simulink model "test_loopback_buf"  (Simulink 6.2)
settings: Solver=ode45  StartTime=0.0  StopTime=4000  RelTol=1e-3
undefined symbols (not defined in the file): Down, Up
libraries: xbsIndex_r3 x1383, xps_library x52, casper_library x37
(part 5 of 8)

== system test_loopback_buf/xaui_buffer_old1 ==
  note: MUX TWO PACKET STREAMS
      | Incomming data is buffered and only stored if it is commited (valid EOF).
      | If a discard command is received, the data is flushed.
  note: THE ACK LINE MUST REMAIN HIGH EVEN WHEN VALID GOES LOW FOR FULL-SPEED READOUT.
      |
      | This is fine for the intended purpose:
      | We read out a full packet at a time, ensuring that ack stays high until EOF is received.
      |
      | this is also important to ensure that the wrong IP address is not used
      | (there is a one-clock delay to fetch the next IP)
  note: PACKET LENGTH SHOULD NOT BE LESS THAN 3 WORDS
  d_in : Inport  Port=1  LatchInput=off
  valid_in : Inport  Port=2  LatchInput=off
  dest_ip_0 : Inport  Port=3  LatchInput=off
  eof_in : Inport  Port=4  LatchInput=off
  discard_in : Inport  Port=5  LatchInput=off
  ack_out : Inport  Port=6  LatchInput=off
  Concat : xbsIndex_r3/Concat  num_inputs=2  explicit_period=off  period=1  dbl_ovrd=off
  Concat3 : xbsIndex_r3/Concat  num_inputs=2  explicit_period=off  period=1  dbl_ovrd=off
  Concat_status : xbsIndex_r3/Concat  num_inputs=4  explicit_period=on  period=1  dbl_ovrd=off
  Constant13 : xbsIndex_r3/Constant  const=0  equ=P=C  arith_type=Boolean  n_bits=1  bin_pt=0  opselect=C  inp2=PCIN>>17  opr=+  inp1=P  carry=CIN  iostate=0  explicit_period=on  period=1  dbl_ovrd=off
  Constant7 : xbsIndex_r3/Constant  const=0  equ=P=C  arith_type=Unsigned  n_bits=32-9  bin_pt=0  opselect=C  inp2=PCIN>>17  opr=+  inp1=P  carry=CIN  iostate=0  explicit_period=on  period=1  dbl_ovrd=off
  Constant9 : xbsIndex_r3/Constant  const=0  equ=P=C  arith_type=Boolean  n_bits=1  bin_pt=0  opselect=C  inp2=PCIN>>17  opr=+  inp1=P  carry=CIN  iostate=0  explicit_period=on  period=1  dbl_ovrd=off
  Convert{,2..4} (4 alike) : xbsIndex_r3/Convert  arith_type=Boolean  n_bits=8  bin_pt=6  quantization=Truncate  overflow=Wrap  latency=0  explicit_period=on  period=1  dbl_ovrd=off  show_param=off  inserted_by_tool=off  pipeline=off
      settings: xl_area=[0, 0, 0, 0, 0, 0, 0]
  Convert{1,5,8..9} (4 alike) : xbsIndex_r3/Convert  arith_type=Unsigned  n_bits=1  bin_pt=0  quantization=Truncate  overflow=Wrap  latency=0  explicit_period=off  period=1  dbl_ovrd=off  show_param=off  inserted_by_tool=off  pipeline=off
      settings: xl_area=[0, 0, 0, 0, 0, 0, 0]
  Gateway Out{1..3,6..8,14,22..25,27..31,39..42} (20 alike) : xbsIndex_r3/Gateway Out  output_type=Double  nbits=8  bin_pt=6  arith_type=Boolean  quantization=Truncate  overflow=Wrap  hdl_port=on  timing_constraint=None  locs_specified=off  LOCs={}  needs_fixed_name=off  show_param=off
      settings: xl_area=[0, 0, 0, 0, 0, 0, 0]
  Inverter4 : xbsIndex_r3/Inverter  latency=0  explicit_period=off  period=1  en=off  dbl_ovrd=off  show_param=off
      settings: xl_area=[0, 0, 0, 0, 0, 0, 0]
  Reinterpret : xbsIndex_r3/Reinterpret  force_arith_type=on  arith_type=Unsigned  force_bin_pt=on  bin_pt=0  force_valid=on
  buf_data3 : xbsIndex_r3/Slice  mode=Lower Bit Location + Width  nbits=64  bit1=33  base1=LSB of Input  bit0=0  base0=LSB of Input  boolean_output=off  explicit_period=off  period=1  dbl_ovrd=off
  buf_eof1 : xbsIndex_r3/Slice  mode=Upper Bit Location + Width  nbits=1  bit1=64  base1=LSB of Input  bit0=0  base0=LSB of Input  boolean_output=on  explicit_period=off  period=1  dbl_ovrd=off
  buf_eof3 : xbsIndex_r3/Slice  mode=Upper Bit Location + Width  nbits=1  bit1=64  base1=LSB of Input  bit0=0  base0=LSB of Input  boolean_output=on  explicit_period=off  period=1  dbl_ovrd=off
  commit : xbsIndex_r3/Logical  logical_function=AND  inputs=2  precision=Full  arith_type=Unsigned  n_bits=8  bin_pt=2  align_bp=on  latency=0  explicit_period=off  period=1  en=off  dbl_ovrd=off  show_param=off
      settings: xl_area=[0, 0, 0, 0, 0, 0, 0]
  data_FWFT : Subsystem  mask{depth_bits=depth_data_bits}
      mask prompts: depth_bits "Fifo Depth (2^?):"
      mask help: A rollback fifo behaves as a normal fifo, except that data which are written in have to be "committed" before they become available for readout. Moreover, any data which are written in and have not been committed can be "discarded", and will never be made available for readout.
      mask init:
      | fmtstr = sprintf('Depth: %d', 2^depth_bits);
      | set_param(gcb, 'AttributesFormatString', fmtstr);
      settings: AttributesFormatString=Depth: 1024
  data_debug : Scope  NumInputPorts=10
      settings: YMin=12000~0~9500~0~15500~0~0~-5~-5~-5  YMax=13300~1~10500~1~17250~1~1~5~5~5  SaveName=ScopeData8
  fifo_empty : xbsIndex_r3/Logical  logical_function=AND  inputs=2  precision=Full  arith_type=Unsigned  n_bits=8  bin_pt=2  align_bp=on  latency=0  explicit_period=off  period=1  en=off  dbl_ovrd=off  show_param=off
      settings: xl_area=[0, 0, 0, 0, 0, 0, 0]
  fifo_full : xbsIndex_r3/Logical  logical_function=OR  inputs=2  precision=Full  arith_type=Unsigned  n_bits=8  bin_pt=2  align_bp=on  latency=0  explicit_period=off  period=1  en=off  dbl_ovrd=off  show_param=off
      settings: xl_area=[0, 0, 0, 0, 0, 0, 0]
  ip_debug : Scope  NumInputPorts=6
      settings: YMin=100~0~0~100~0~-5  YMax=103~1~1~103~1~5  SaveName=ScopeData9
  ip_fifo : Subsystem  mask{depth_bits=depth_hdr_bits}
      mask prompts: depth_bits "Fifo Depth (2^?):"
      mask help: A rollback fifo behaves as a normal fifo, except that data which are written in have to be "committed" before they become available for readout. Moreover, any data which are written in and have not been committed can be "discarded", and will never be made available for readout.
      mask init:
      | fmtstr = sprintf('Depth: %d', 2^depth_bits);
      | set_param(gcb, 'AttributesFormatString', fmtstr);
      settings: AttributesFormatString=Depth: 256
  overflow_cnt : xps_library/software register  Tag=xps:sw_reg  io_dir=To Processor  arith_type=Unsigned  bitwidth=32  bin_pt=0  sample_period=1  gw_name=test_loopback_buf_xaui_buffer_old1_overflow_cnt_user_data_in
  overflows : xbsIndex_r3/Counter  cnt_type=Free Running  n_bits=32  bin_pt=0  arith_type=Unsigned  start_count=0  cnt_to=Inf  cnt_by_val=1  operation=Up  explicit_period=off  period=1  load_pin=off  rst=off  en=on  dbl_ovrd=off  show_param=off  use_rpm=on  gen_core=off
      settings: xl_area=[0, 0, 0, 0, 0, 0, 0]
  status : xps_library/software register  Tag=xps:sw_reg  io_dir=To Processor  arith_type=Unsigned  bitwidth=32  bin_pt=0  sample_period=1  gw_name=test_loopback_buf_xaui_buffer_old1_status_user_data_in
  status1 : Scope  NumInputPorts=4
      settings: YMin=-1~-1~-1~-1  YMax=1~1~1~1  SaveName=ScopeData6
  valid_eof_0 : xbsIndex_r3/Logical  logical_function=AND  inputs=2  precision=Full  arith_type=Unsigned  n_bits=8  bin_pt=2  align_bp=on  latency=0  explicit_period=on  period=1  en=off  dbl_ovrd=off  show_param=off
      settings: xl_area=[0, 0, 0, 0, 0, 0, 0]
  data : Outport
  valid : Outport  Port=2
  ip_addr : Outport  Port=3
  eof : Outport  Port=4
  discard : Outport  Port=5
  buffer_overflow : Outport  Port=6
  buffer_empty : Outport  Port=7
  ack_in : Outport  Port=8
  status_out : Outport  Port=9
  wires:
  Constant13/1 -> discard/1
  fifo_full/1 -> buffer_overflow/1, overflows/1
  fifo_empty/1 -> buffer_empty/1
  [ip_empty] -> fifo_empty/1
  [data_empty] -> fifo_empty/2
  [ip_full] -> fifo_full/1
  [data_full] -> fifo_full/2
  [ip_full] -> Convert1/1, Gateway Out7/1
  [data_full] -> Gateway Out8/1, Convert5/1
  [ip_empty] -> Convert8/1, Gateway Out6/1
  [data_empty] -> Convert9/1, Gateway Out14/1
  Concat_status/1 -> Concat3/2, status_out/1
  Concat3/1 -> status/1
  Constant7/1 -> Concat3/1
  discard_in/1 -> Convert3/1
  Concat/1 -> data_FWFT/1(din)
  data_FWFT/4(full) -> [data_full]
  ip_fifo/3(full) -> [ip_full]
  commit/1 -> ip_fifo/3(commit), ip_fifo/2(we), [ip_commit]
  d_in/1 -> Reinterpret/1
  valid_in/1 -> Convert/1
  dest_ip_0/1 -> ip_fifo/1(din), [ip_in]
  eof_in/1 -> Convert2/1
  data_FWFT/3(wr_ack) -> ack_in/1
  ip_fifo/4(empty) -> [ip_empty]
  Inverter4/1 -> commit/2
  valid_eof_0/1 -> Concat/1, [in_valid_eof], data_FWFT/3(commit)
  data_FWFT/1(dout) -> buf_eof1/1, buf_eof3/1, buf_data3/1
  data_FWFT/2(valid) -> valid/1, [v_out]
  ip_fifo/1(dout) -> ip_addr/1, [ip_out]
  Constant9/1 -> ip_fifo/4(discard)
  overflows/1 -> overflow_cnt/1
  Gateway Out24/1 -> data_debug/1
  Gateway Out22/1 -> data_debug/2
  Gateway Out23/1 -> data_debug/3
  Gateway Out25/1 -> data_debug/4
  Gateway Out29/1 -> ip_debug/1
  Gateway Out27/1 -> ip_debug/2
  Gateway Out28/1 -> ip_debug/3
  Gateway Out30/1 -> ip_debug/4
  Gateway Out31/1 -> ip_debug/5
  Gateway Out39/1 -> data_debug/5
  Gateway Out41/1 -> data_debug/6
  Gateway Out40/1 -> data_debug/7
  Gateway Out42/1 -> ip_debug/6
  data_FWFT/5(empty) -> [data_empty]
  buf_data3/1 -> data/1, [d_out]
  buf_eof3/1 -> eof/1, [eof_out]
  [in_valid_eof] -> commit/1
  Gateway Out7/1 -> status1/1
  Gateway Out8/1 -> status1/2
  Gateway Out6/1 -> status1/3
  Gateway Out14/1 -> status1/4
  Convert1/1 -> Concat_status/1
  Convert5/1 -> Concat_status/2
  Convert8/1 -> Concat_status/3
  Convert9/1 -> Concat_status/4
  Gateway Out1/1 -> data_debug/8
  [ip_out] -> Gateway Out1/1
  [eof_out] -> Gateway Out40/1
  [v_out] -> Gateway Out41/1
  [d_out] -> Gateway Out39/1
  [ip_in] -> Gateway Out25/1
  [d_in] -> Gateway Out24/1
  [v_in] -> Gateway Out22/1
  [in_valid_eof] -> Gateway Out23/1
  [ip_in] -> Gateway Out29/1
  [ip_out] -> Gateway Out30/1
  [eof_out] -> Gateway Out31/1
  ack_out/1 -> Convert4/1
  [data_ack] -> Gateway Out42/1
  [ip_commit] -> Gateway Out27/1
  [data_full] -> Inverter4/1
  [ip_fetch] -> Gateway Out28/1
  [data_ack] -> data_FWFT/5(ack)
  Gateway Out2/1 -> data_debug/9
  [data_ack] -> Gateway Out2/1
  buf_eof1/1 -> [ip_fetch]
  [ip_fetch] -> ip_fifo/5(fetch)
  Reinterpret/1 -> Concat/2, [d_in]
  Convert/1 -> valid_eof_0/1, data_FWFT/2(we), [v_in]
  Convert2/1 -> valid_eof_0/2
  Convert3/1 -> data_FWFT/4(discard)
  Convert4/1 -> [data_ack]
  Gateway Out3/1 -> data_debug/10
  [data_full] -> Gateway Out3/1

== system test_loopback_buf/loopback/fwft_fifo ==
  din : Inport  Port=1  LatchInput=off
  we : Inport  Port=2  LatchInput=off
  ack : Inport  Port=3  LatchInput=off
  Convert : xbsIndex_r3/Convert  Orientation=left  arith_type=Boolean  n_bits=1  bin_pt=0  quantization=Truncate  overflow=Wrap  latency=0  explicit_period=off  period=1  dbl_ovrd=off  show_param=off  inserted_by_tool=off  pipeline=off
      settings: xl_area=[0, 0, 0, 0, 0, 0, 0]
  FIFO : xbsIndex_r3/FIFO  depth=256  percent_nbits=1  store_only_valid=on  init_zero=on  explicit_period=off  period=1  rst=off  en=off  use_almost_empty=off  almost_empty_offset=6  use_almost_full=off  almost_full_offset=6  dbl_ovrd=off  show_param=off  mem_type=Block RAM  gen_core=off
      settings: xl_area=[0, 0, 0, 0, 0, 0, 0]
  Inverter1 : xbsIndex_r3/Inverter  latency=0  explicit_period=off  period=1  en=off  dbl_ovrd=off  show_param=off
      settings: xl_area=[0, 0, 0, 0, 0, 0, 0]
  Logical1 : xbsIndex_r3/Logical  logical_function=OR  inputs=2  precision=Full  arith_type=Unsigned  n_bits=8  bin_pt=2  align_bp=on  latency=0  explicit_period=off  period=1  en=off  dbl_ovrd=off  show_param=off
      settings: xl_area=[0, 0, 0, 0, 0, 0, 0]
  Register2 : xbsIndex_r3/Register  init=0  reg_only_valid=off  explicit_period=on  period=1  rst=off  en=on  out_en=off  dbl_ovrd=off  show_param=off
      settings: xl_area=[0, 0, 0, 0, 0, 0, 0]
  dout : Outport
  valid : Outport  Port=2
  wires:
  din/1 -> FIFO/1
  we/1 -> FIFO/2
  FIFO/1 -> dout/1
  FIFO/2 -> Register2/1
  Logical1/1 -> FIFO/3, Register2/2
  ack/1 -> Logical1/1
  Register2/1 -> Convert/1, Inverter1/1
  Convert/1 -> Logical1/2
  Inverter1/1 -> valid/1

== system test_loopback_buf/loopback/rollback_fifo ==
  din : Inport  Port=1  LatchInput=off
  we : Inport  Orientation=left  Port=2  LatchInput=off
  commit : Inport  Port=3  LatchInput=off
  discard : Inport  Port=4  LatchInput=off
  re : Inport  Port=5  LatchInput=off
  Constant5 : xbsIndex_r3/Constant  const=0  equ=P=C  arith_type=Boolean  n_bits=1  bin_pt=0  opselect=C  inp2=PCIN>>17  opr=+  inp1=P  carry=CIN  iostate=0  explicit_period=on  period=1  dbl_ovrd=off
  Delay1 : xbsIndex_r3/Delay  latency=1  reg_retiming=off  explicit_period=off  period=1  en=off  accept_only_valid=off  init_zero=on  dbl_ovrd=off  show_param=off
      settings: xl_area=[0, 0, 0, 0, 0, 0, 0]
  Dual Port RAM : xbsIndex_r3/Dual Port RAM  depth=2^depth_bits  initVector=0  write_mode_A=Read Before Write  write_mode_B=Read Before Write  latency=1  mem_collision=off  init_zero=on  explicit_period=off  period=1  dbl_ovrd=off  rst_a=off  init_a=0  rst_b=off  init_b=0  show_param=off  distributed_mem=off  use_rpm=off  gen_core=off
      settings: xl_area=[0, 0, 0, 0, 0, 0, 0]
  Inverter1 : xbsIndex_r3/Inverter  latency=0  explicit_period=off  period=1  en=off  dbl_ovrd=off  show_param=off
      settings: xl_area=[0, 0, 0, 0, 0, 0, 0]
  Inverter2 : xbsIndex_r3/Inverter  Orientation=up  latency=0  explicit_period=off  period=1  en=off  dbl_ovrd=off  show_param=off
      settings: xl_area=[0, 0, 0, 0, 0, 0, 0]
  Logical1 : xbsIndex_r3/Logical  logical_function=AND  inputs=2  precision=Full  arith_type=Unsigned  n_bits=8  bin_pt=2  align_bp=on  latency=0  explicit_period=off  period=1  en=off  dbl_ovrd=off  show_param=off
      settings: xl_area=[0, 0, 0, 0, 0, 0, 0]
  Logical3 : xbsIndex_r3/Logical  Orientation=left  logical_function=AND  inputs=2  precision=Full  arith_type=Unsigned  n_bits=8  bin_pt=2  align_bp=on  latency=0  explicit_period=off  period=1  en=off  dbl_ovrd=off  show_param=off
      settings: xl_area=[0, 0, 0, 0, 0, 0, 0]
  Logical4 : xbsIndex_r3/Logical  logical_function=AND  inputs=2  precision=Full  arith_type=Unsigned  n_bits=8  bin_pt=2  align_bp=on  latency=0  explicit_period=off  period=1  en=off  dbl_ovrd=off  show_param=off
      settings: xl_area=[0, 0, 0, 0, 0, 0, 0]
  Logical5 : xbsIndex_r3/Logical  logical_function=XOR  inputs=2  precision=Full  arith_type=Unsigned  n_bits=8  bin_pt=2  align_bp=on  latency=0  explicit_period=off  period=1  en=off  dbl_ovrd=off  show_param=off
      settings: xl_area=[0, 0, 0, 0, 0, 0, 0]
  Logical6 : xbsIndex_r3/Logical  logical_function=AND  inputs=2  precision=Full  arith_type=Unsigned  n_bits=8  bin_pt=2  align_bp=on  latency=0  explicit_period=off  period=1  en=off  dbl_ovrd=off  show_param=off
      settings: xl_area=[0, 0, 0, 0, 0, 0, 0]
  Relational1 : xbsIndex_r3/Relational  mode=a=b  latency=0  explicit_period=on  period=1  en=off  dbl_ovrd=off  show_param=off
      settings: xl_area=[0, 0, 0, 0, 0, 0, 0]
  Relational2 : xbsIndex_r3/Relational  mode=a=b  latency=0  explicit_period=on  period=1  en=off  dbl_ovrd=off  show_param=off
      settings: xl_area=[0, 0, 0, 0, 0, 0, 0]
  Slice : xbsIndex_r3/Slice  mode=Two Bit Locations  nbits=1  bit1=-1  base1=MSB of Input  bit0=0  base0=LSB of Input  boolean_output=off  explicit_period=off  period=1  dbl_ovrd=off
  Slice1 : xbsIndex_r3/Slice  mode=Upper Bit Location + Width  nbits=1  bit1=0  base1=MSB of Input  bit0=0  base0=LSB of Input  boolean_output=on  explicit_period=off  period=1  dbl_ovrd=off
  Slice2 : xbsIndex_r3/Slice  mode=Two Bit Locations  nbits=1  bit1=-1  base1=MSB of Input  bit0=0  base0=LSB of Input  boolean_output=off  explicit_period=off  period=1  dbl_ovrd=off
  Slice3 : xbsIndex_r3/Slice  mode=Upper Bit Location + Width  nbits=1  bit1=0  base1=MSB of Input  bit0=0  base0=LSB of Input  boolean_output=on  explicit_period=off  period=1  dbl_ovrd=off
  rd_cnt : xbsIndex_r3/Counter  cnt_type=Free Running  n_bits=depth_bits + 1  bin_pt=0  arith_type=Unsigned  start_count=0  cnt_to=Inf  cnt_by_val=1  operation=Up  explicit_period=on  period=1  load_pin=off  rst=off  en=on  dbl_ovrd=off  show_param=off  use_rpm=on  gen_core=off
      settings: xl_area=[0, 0, 0, 0, 0, 0, 0]
  set_cnt : Subsystem
  dout : Outport
  valid : Outport  Port=2
  wr_ack : Outport  Orientation=left  Port=3
  full : Outport  Port=4
  empty : Outport  Port=5
  wires:
  Relational2/1 -> Logical1/1
  Logical6/1 -> Inverter2/1, full/1
  Logical5/1 -> Logical6/1
  Relational1/1 -> Logical6/2
  Slice1/1 -> Logical5/2
  Slice3/1 -> Logical5/1
  Slice2/1 -> Relational1/1, Dual Port RAM/1
  din/1 -> Dual Port RAM/2, Dual Port RAM/5
  Slice/1 -> Relational1/2, Dual Port RAM/4
  set_cnt/2(cnt) -> Slice2/1, Slice3/1
  set_cnt/1(set_cnt) -> Relational2/1
  rd_cnt/1 -> Relational2/2, Slice1/1, Slice/1
  commit/1 -> set_cnt/1(set)
  Inverter2/1 -> Logical1/2, Logical3/1
  we/1 -> Logical3/2
  Logical3/1 -> wr_ack/1, Dual Port RAM/3, set_cnt/3(en)
  discard/1 -> set_cnt/2(undo)
  Constant5/1 -> Dual Port RAM/6
  Dual Port RAM/2 -> dout/1
  Logical1/1 -> Inverter1/1, empty/1
  Inverter1/1 -> Logical4/2
  re/1 -> Logical4/1
  Logical4/1 -> rd_cnt/1, Delay1/1
  Delay1/1 -> valid/1

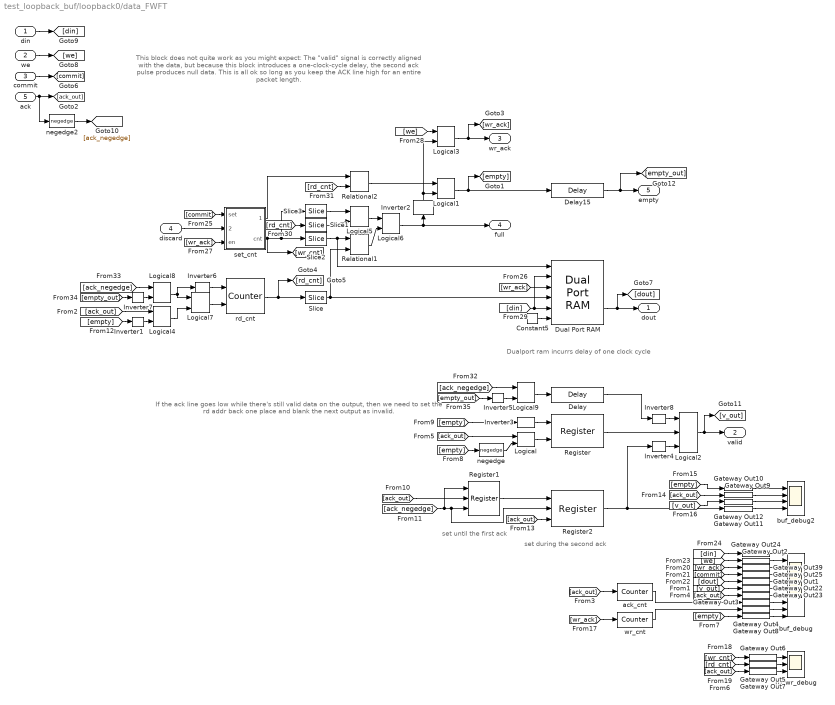
== system test_loopback_buf/loopback0/data_FWFT ==
  note: This block does not quite work as you might expect:
      | The "valid" signal is correctly aligned with the data,
      | but because this block introduces a one-clock-cycle delay,
      | the second ack pulse produces null data.
      |
      | This is all ok so long as you keep the ACK line high for an entire packet length.
  note: set until the first ack
  note: set during the second ack
  note: If the ack line goes low while there's still valid data on the output,
      | then we need to set the rd addr back one place and blank the next
      | output as invalid.
  note: Dualport ram incurrs delay
      | of one clock cycle
  din : Inport  Port=1  LatchInput=off
  we : Inport  Port=2  LatchInput=off
  commit : Inport  Port=3  LatchInput=off
  discard : Inport  Port=4  LatchInput=off
  ack : Inport  Port=5  LatchInput=off
  Constant5 : xbsIndex_r3/Constant  const=0  equ=P=C  arith_type=Boolean  n_bits=1  bin_pt=0  opselect=C  inp2=PCIN>>17  opr=+  inp1=P  carry=CIN  iostate=0  explicit_period=on  period=1  dbl_ovrd=off
  Delay : xbsIndex_r3/Delay  latency=1  reg_retiming=on  explicit_period=off  period=1  en=off  accept_only_valid=off  init_zero=on  dbl_ovrd=off  show_param=off
      settings: xl_area=[0, 0, 0, 0, 0, 0, 0]
  Delay15 : xbsIndex_r3/Delay  latency=1  reg_retiming=on  explicit_period=off  period=1  en=off  accept_only_valid=off  init_zero=on  dbl_ovrd=off  show_param=off
      settings: xl_area=[0, 0, 0, 0, 0, 0, 0]
  Dual Port RAM : xbsIndex_r3/Dual Port RAM  depth=2^depth_bits  initVector=0  write_mode_A=Read Before Write  write_mode_B=Read Before Write  latency=1  mem_collision=off  init_zero=on  explicit_period=off  period=1  dbl_ovrd=off  rst_a=off  init_a=0  rst_b=off  init_b=0  show_param=off  distributed_mem=off  use_rpm=off  gen_core=off
      settings: xl_area=[0, 0, 0, 0, 0, 0, 0]
  Gateway Out{1..12,22..25,39} (17 alike) : xbsIndex_r3/Gateway Out  output_type=Double  nbits=8  bin_pt=6  arith_type=Boolean  quantization=Truncate  overflow=Wrap  hdl_port=on  timing_constraint=None  locs_specified=off  LOCs={}  needs_fixed_name=off  show_param=off
      settings: xl_area=[0, 0, 0, 0, 0, 0, 0]
  Inverter{1,3..8} (7 alike) : xbsIndex_r3/Inverter  latency=0  explicit_period=off  period=1  en=off  dbl_ovrd=off  show_param=off
      settings: xl_area=[0, 0, 0, 0, 0, 0, 0]
  Inverter2 : xbsIndex_r3/Inverter  Orientation=up  latency=0  explicit_period=off  period=1  en=off  dbl_ovrd=off  show_param=off
      settings: xl_area=[0, 0, 0, 0, 0, 0, 0]
  Logical : xbsIndex_r3/Logical  logical_function=OR  inputs=2  precision=Full  arith_type=Unsigned  n_bits=8  bin_pt=2  align_bp=on  latency=0  explicit_period=off  period=1  en=off  dbl_ovrd=off  show_param=off
      settings: xl_area=[0, 0, 0, 0, 0, 0, 0]
  Logical1 : xbsIndex_r3/Logical  logical_function=AND  inputs=2  precision=Full  arith_type=Unsigned  n_bits=8  bin_pt=2  align_bp=on  latency=0  explicit_period=on  period=1  en=off  dbl_ovrd=off  show_param=off
      settings: xl_area=[0, 0, 0, 0, 0, 0, 0]
  Logical2 : xbsIndex_r3/Logical  logical_function=AND  inputs=3  precision=Full  arith_type=Unsigned  n_bits=8  bin_pt=2  align_bp=on  latency=0  explicit_period=on  period=1  en=off  dbl_ovrd=off  show_param=off
      settings: xl_area=[0, 0, 0, 0, 0, 0, 0]
  Logical{3..4,6,8..9} (5 alike) : xbsIndex_r3/Logical  logical_function=AND  inputs=2  precision=Full  arith_type=Unsigned  n_bits=8  bin_pt=2  align_bp=on  latency=0  explicit_period=off  period=1  en=off  dbl_ovrd=off  show_param=off
      settings: xl_area=[0, 0, 0, 0, 0, 0, 0]
  Logical5 : xbsIndex_r3/Logical  logical_function=XOR  inputs=2  precision=Full  arith_type=Unsigned  n_bits=8  bin_pt=2  align_bp=on  latency=0  explicit_period=off  period=1  en=off  dbl_ovrd=off  show_param=off
      settings: xl_area=[0, 0, 0, 0, 0, 0, 0]
  Logical7 : xbsIndex_r3/Logical  logical_function=OR  inputs=2  precision=Full  arith_type=Unsigned  n_bits=8  bin_pt=2  align_bp=on  latency=0  explicit_period=off  period=1  en=off  dbl_ovrd=off  show_param=off
      settings: xl_area=[0, 0, 0, 0, 0, 0, 0]
  Register : xbsIndex_r3/Register  init=0  reg_only_valid=off  explicit_period=on  period=1  rst=off  en=on  out_en=off  dbl_ovrd=off  show_param=off
      settings: xl_area=[0, 0, 0, 0, 0, 0, 0]
  Register1 : xbsIndex_r3/Register  init=0  reg_only_valid=off  explicit_period=on  period=1  rst=on  en=on  out_en=off  dbl_ovrd=off  show_param=off
      settings: xl_area=[0, 0, 0, 0, 0, 0, 0]
  Register2 : xbsIndex_r3/Register  init=0  reg_only_valid=off  explicit_period=on  period=1  rst=on  en=on  out_en=off  dbl_ovrd=off  show_param=off
      settings: xl_area=[0, 0, 0, 0, 0, 0, 0]
  Relational1 : xbsIndex_r3/Relational  mode=a=b  latency=0  explicit_period=on  period=1  en=off  dbl_ovrd=off  show_param=off
      settings: xl_area=[0, 0, 0, 0, 0, 0, 0]
  Relational2 : xbsIndex_r3/Relational  mode=a=b  latency=0  explicit_period=on  period=1  en=off  dbl_ovrd=off  show_param=off
      settings: xl_area=[0, 0, 0, 0, 0, 0, 0]
  Slice : xbsIndex_r3/Slice  mode=Two Bit Locations  nbits=1  bit1=-1  base1=MSB of Input  bit0=0  base0=LSB of Input  boolean_output=off  explicit_period=off  period=1  dbl_ovrd=off
  Slice1 : xbsIndex_r3/Slice  mode=Upper Bit Location + Width  nbits=1  bit1=0  base1=MSB of Input  bit0=0  base0=LSB of Input  boolean_output=on  explicit_period=off  period=1  dbl_ovrd=off
  Slice2 : xbsIndex_r3/Slice  mode=Two Bit Locations  nbits=1  bit1=-1  base1=MSB of Input  bit0=0  base0=LSB of Input  boolean_output=off  explicit_period=off  period=1  dbl_ovrd=off
  Slice3 : xbsIndex_r3/Slice  mode=Upper Bit Location + Width  nbits=1  bit1=0  base1=MSB of Input  bit0=0  base0=LSB of Input  boolean_output=on  explicit_period=off  period=1  dbl_ovrd=off
  ack_cnt : xbsIndex_r3/Counter  cnt_type=Free Running  n_bits=depth_bits + 1  bin_pt=0  arith_type=Unsigned  start_count=0  cnt_to=Inf  cnt_by_val=1  operation=Up  explicit_period=on  period=1  load_pin=off  rst=off  en=on  dbl_ovrd=off  show_param=off  use_rpm=on  gen_core=off
      settings: xl_area=[0, 0, 0, 0, 0, 0, 0]
  buf_debug : Scope  NumInputPorts=10
      settings: YMin=12000~0~9500~0~15500~-5~-5~-5~-5~-5  YMax=13300~1~10500~1~17250~5~5~5~5~5  SaveName=ScopeData13
  buf_debug2 : Scope  NumInputPorts=4
      settings: YMin=0~1~0~-1  YMax=1~1~1~1  SaveName=ScopeData15
  negedge : casper_library/Misc/negedge  Tag=Rising Edge Detector
  negedge2 : casper_library/Misc/negedge  Tag=Rising Edge Detector
  rd_cnt : xbsIndex_r3/Counter  cnt_type=Free Running  n_bits=depth_bits + 1  bin_pt=0  arith_type=Unsigned  start_count=0  cnt_to=Inf  cnt_by_val=1  operation=Up/Down  explicit_period=on  period=1  load_pin=off  rst=off  en=on  dbl_ovrd=off  show_param=off  use_rpm=on  gen_core=off
      settings: xl_area=[0, 0, 0, 0, 0, 0, 0]
  rd_wr_debug : Scope  NumInputPorts=3
      settings: YMin=12000~0~-5  YMax=13300~1~5  SaveName=ScopeData14
  set_cnt : Subsystem
  wr_cnt : xbsIndex_r3/Counter  cnt_type=Free Running  n_bits=depth_bits + 1  bin_pt=0  arith_type=Unsigned  start_count=0  cnt_to=Inf  cnt_by_val=1  operation=Up  explicit_period=on  period=1  load_pin=off  rst=off  en=on  dbl_ovrd=off  show_param=off  use_rpm=on  gen_core=off
      settings: xl_area=[0, 0, 0, 0, 0, 0, 0]
  dout : Outport
  valid : Outport  Port=2
  wr_ack : Outport  Port=3
  full : Outport  Port=4
  empty : Outport  Port=5
  wires:
  Relational2/1 -> Logical1/1
  Logical6/1 -> Inverter2/1, full/1
  Logical5/1 -> Logical6/1
  Relational1/1 -> Logical6/2
  Slice1/1 -> Logical5/2
  Slice3/1 -> Logical5/1
  Slice2/1 -> Relational1/1, Dual Port RAM/1
  Slice/1 -> Relational1/2, Dual Port RAM/4
  set_cnt/2(cnt) -> Slice3/1, Slice2/1, [wr_cnt]
  set_cnt/1(set_cnt) -> Relational2/1
  rd_cnt/1 -> [rd_cnt], Slice/1
  commit/1 -> [commit]
  Inverter2/1 -> Logical1/2, Logical3/2
  we/1 -> [we]
  discard/1 -> set_cnt/2(undo)
  Constant5/1 -> Dual Port RAM/6
  Dual Port RAM/2 -> dout/1, [dout]
  Logical1/1 -> [empty], Delay15/1
  Gateway Out24/1 -> buf_debug/1
  Gateway Out2/1 -> buf_debug/2
  Gateway Out39/1 -> buf_debug/3
  Gateway Out25/1 -> buf_debug/4
  Gateway Out1/1 -> buf_debug/5
  Gateway Out22/1 -> buf_debug/6
  Gateway Out23/1 -> buf_debug/7
  Gateway Out3/1 -> buf_debug/8
  Gateway Out4/1 -> buf_debug/9
  ack_cnt/1 -> Gateway Out3/1
  wr_cnt/1 -> Gateway Out4/1
  [empty] -> Inverter1/1
  [v_out] -> Gateway Out22/1
  ack/1 -> [ack_out], negedge2/1
  [ack_out] -> Logical4/1
  [ack_out] -> ack_cnt/1
  [ack_out] -> Gateway Out23/1
  Gateway Out6/1 -> rd_wr_debug/1
  Gateway Out5/1 -> rd_wr_debug/2
  Gateway Out7/1 -> rd_wr_debug/3
  [ack_out] -> Gateway Out7/1
  Gateway Out8/1 -> buf_debug/10
  [empty] -> Gateway Out8/1
  Inverter1/1 -> Logical4/2
  Logical2/1 -> valid/1, [v_out]
  [ack_negedge] -> Register1/1, Register1/3, Register2/2
  [ack_out] -> Register1/2
  Register1/1 -> Register2/1
  Gateway Out10/1 -> buf_debug2/1
  Gateway Out9/1 -> buf_debug2/2
  Gateway Out12/1 -> buf_debug2/3
  Gateway Out11/1 -> buf_debug2/4
  [ack_out] -> Gateway Out9/1
  [empty] -> Gateway Out10/1
  [v_out] -> Gateway Out12/1
  [ack_out] -> Register2/3
  [wr_ack] -> wr_cnt/1
  [wr_cnt] -> Gateway Out6/1
  [rd_cnt] -> Gateway Out5/1
  [wr_ack] -> Gateway Out39/1
  [commit] -> Gateway Out25/1
  [dout] -> Gateway Out1/1
  [we] -> Gateway Out2/1
  [din] -> Gateway Out24/1
  [commit] -> set_cnt/1(set)
  [wr_ack] -> Dual Port RAM/3
  [wr_ack] -> set_cnt/3(en)
  [we] -> Logical3/1
  Logical3/1 -> wr_ack/1, [wr_ack]
  [din] -> Dual Port RAM/2, Dual Port RAM/5
  din/1 -> [din]
  [rd_cnt] -> Slice1/1
  [rd_cnt] -> Relational2/2
  Register2/1 -> Gateway Out11/1, Inverter4/1
  negedge2/1 -> [ack_negedge]
  Inverter6/1 -> rd_cnt/1
  Logical7/1 -> rd_cnt/2
  Logical4/1 -> Logical7/2
  Logical8/1 -> Inverter6/1, Logical7/1
  [ack_negedge] -> Logical8/1
  [empty_out] -> Inverter7/1
  Inverter7/1 -> Logical8/2
  [ack_negedge] -> Logical9/1
  [empty_out] -> Inverter5/1
  Inverter5/1 -> Logical9/2
  Logical9/1 -> Delay/1
  Delay/1 -> Inverter8/1
  Inverter3/1 -> Register/1
  [empty] -> Inverter3/1
  Logical/1 -> Register/2
  [empty] -> negedge/1
  [ack_out] -> Logical/1
  negedge/1 -> Logical/2
  Inverter4/1 -> Logical2/3
  Inverter8/1 -> Logical2/1
  Register/1 -> Logical2/2
  Delay15/1 -> empty/1, [empty_out]

== system test_loopback_buf/loopback1/fwft_fifo ==
  din : Inport  Port=1  LatchInput=off
  we : Inport  Port=2  LatchInput=off
  ack : Inport  Port=3  LatchInput=off
  Convert : xbsIndex_r3/Convert  Orientation=left  arith_type=Boolean  n_bits=1  bin_pt=0  quantization=Truncate  overflow=Wrap  latency=0  explicit_period=off  period=1  dbl_ovrd=off  show_param=off  inserted_by_tool=off  pipeline=off
      settings: xl_area=[0, 0, 0, 0, 0, 0, 0]
  FIFO : xbsIndex_r3/FIFO  depth=256  percent_nbits=1  store_only_valid=on  init_zero=on  explicit_period=off  period=1  rst=off  en=off  use_almost_empty=off  almost_empty_offset=6  use_almost_full=off  almost_full_offset=6  dbl_ovrd=off  show_param=off  mem_type=Block RAM  gen_core=off
      settings: xl_area=[0, 0, 0, 0, 0, 0, 0]
  Inverter1 : xbsIndex_r3/Inverter  latency=0  explicit_period=off  period=1  en=off  dbl_ovrd=off  show_param=off
      settings: xl_area=[0, 0, 0, 0, 0, 0, 0]
  Logical1 : xbsIndex_r3/Logical  logical_function=OR  inputs=2  precision=Full  arith_type=Unsigned  n_bits=8  bin_pt=2  align_bp=on  latency=0  explicit_period=off  period=1  en=off  dbl_ovrd=off  show_param=off
      settings: xl_area=[0, 0, 0, 0, 0, 0, 0]
  Register2 : xbsIndex_r3/Register  init=0  reg_only_valid=off  explicit_period=on  period=1  rst=off  en=on  out_en=off  dbl_ovrd=off  show_param=off
      settings: xl_area=[0, 0, 0, 0, 0, 0, 0]
  dout : Outport
  valid : Outport  Port=2
  wires:
  Inverter1/1 -> valid/1
  Convert/1 -> Logical1/2
  Register2/1 -> Inverter1/1, Convert/1
  ack/1 -> Logical1/1
  Logical1/1 -> Register2/2, FIFO/3
  FIFO/2 -> Register2/1
  FIFO/1 -> dout/1
  we/1 -> FIFO/2
  din/1 -> FIFO/1

== system test_loopback_buf/loopback1/rollback_fifo ==
  din : Inport  Port=1  LatchInput=off
  we : Inport  Orientation=left  Port=2  LatchInput=off
  commit : Inport  Port=3  LatchInput=off
  discard : Inport  Port=4  LatchInput=off
  re : Inport  Port=5  LatchInput=off
  Constant5 : xbsIndex_r3/Constant  const=0  equ=P=C  arith_type=Boolean  n_bits=1  bin_pt=0  opselect=C  inp2=PCIN>>17  opr=+  inp1=P  carry=CIN  iostate=0  explicit_period=on  period=1  dbl_ovrd=off
  Delay1 : xbsIndex_r3/Delay  latency=1  reg_retiming=off  explicit_period=off  period=1  en=off  accept_only_valid=off  init_zero=on  dbl_ovrd=off  show_param=off
      settings: xl_area=[0, 0, 0, 0, 0, 0, 0]
  Dual Port RAM : xbsIndex_r3/Dual Port RAM  depth=2^depth_bits  initVector=0  write_mode_A=Read Before Write  write_mode_B=Read Before Write  latency=1  mem_collision=off  init_zero=on  explicit_period=off  period=1  dbl_ovrd=off  rst_a=off  init_a=0  rst_b=off  init_b=0  show_param=off  distributed_mem=off  use_rpm=off  gen_core=off
      settings: xl_area=[0, 0, 0, 0, 0, 0, 0]
  Inverter1 : xbsIndex_r3/Inverter  latency=0  explicit_period=off  period=1  en=off  dbl_ovrd=off  show_param=off
      settings: xl_area=[0, 0, 0, 0, 0, 0, 0]
  Inverter2 : xbsIndex_r3/Inverter  Orientation=up  latency=0  explicit_period=off  period=1  en=off  dbl_ovrd=off  show_param=off
      settings: xl_area=[0, 0, 0, 0, 0, 0, 0]
  Logical1 : xbsIndex_r3/Logical  logical_function=AND  inputs=2  precision=Full  arith_type=Unsigned  n_bits=8  bin_pt=2  align_bp=on  latency=0  explicit_period=off  period=1  en=off  dbl_ovrd=off  show_param=off
      settings: xl_area=[0, 0, 0, 0, 0, 0, 0]
  Logical3 : xbsIndex_r3/Logical  Orientation=left  logical_function=AND  inputs=2  precision=Full  arith_type=Unsigned  n_bits=8  bin_pt=2  align_bp=on  latency=0  explicit_period=off  period=1  en=off  dbl_ovrd=off  show_param=off
      settings: xl_area=[0, 0, 0, 0, 0, 0, 0]
  Logical4 : xbsIndex_r3/Logical  logical_function=AND  inputs=2  precision=Full  arith_type=Unsigned  n_bits=8  bin_pt=2  align_bp=on  latency=0  explicit_period=off  period=1  en=off  dbl_ovrd=off  show_param=off
      settings: xl_area=[0, 0, 0, 0, 0, 0, 0]
  Logical5 : xbsIndex_r3/Logical  logical_function=XOR  inputs=2  precision=Full  arith_type=Unsigned  n_bits=8  bin_pt=2  align_bp=on  latency=0  explicit_period=off  period=1  en=off  dbl_ovrd=off  show_param=off
      settings: xl_area=[0, 0, 0, 0, 0, 0, 0]
  Logical6 : xbsIndex_r3/Logical  logical_function=AND  inputs=2  precision=Full  arith_type=Unsigned  n_bits=8  bin_pt=2  align_bp=on  latency=0  explicit_period=off  period=1  en=off  dbl_ovrd=off  show_param=off
      settings: xl_area=[0, 0, 0, 0, 0, 0, 0]
  Relational1 : xbsIndex_r3/Relational  mode=a=b  latency=0  explicit_period=on  period=1  en=off  dbl_ovrd=off  show_param=off
      settings: xl_area=[0, 0, 0, 0, 0, 0, 0]
  Relational2 : xbsIndex_r3/Relational  mode=a=b  latency=0  explicit_period=on  period=1  en=off  dbl_ovrd=off  show_param=off
      settings: xl_area=[0, 0, 0, 0, 0, 0, 0]
  Slice : xbsIndex_r3/Slice  mode=Two Bit Locations  nbits=1  bit1=-1  base1=MSB of Input  bit0=0  base0=LSB of Input  boolean_output=off  explicit_period=off  period=1  dbl_ovrd=off
  Slice1 : xbsIndex_r3/Slice  mode=Upper Bit Location + Width  nbits=1  bit1=0  base1=MSB of Input  bit0=0  base0=LSB of Input  boolean_output=on  explicit_period=off  period=1  dbl_ovrd=off
  Slice2 : xbsIndex_r3/Slice  mode=Two Bit Locations  nbits=1  bit1=-1  base1=MSB of Input  bit0=0  base0=LSB of Input  boolean_output=off  explicit_period=off  period=1  dbl_ovrd=off
  Slice3 : xbsIndex_r3/Slice  mode=Upper Bit Location + Width  nbits=1  bit1=0  base1=MSB of Input  bit0=0  base0=LSB of Input  boolean_output=on  explicit_period=off  period=1  dbl_ovrd=off
  rd_cnt : xbsIndex_r3/Counter  cnt_type=Free Running  n_bits=depth_bits + 1  bin_pt=0  arith_type=Unsigned  start_count=0  cnt_to=Inf  cnt_by_val=1  operation=Up  explicit_period=on  period=1  load_pin=off  rst=off  en=on  dbl_ovrd=off  show_param=off  use_rpm=on  gen_core=off
      settings: xl_area=[0, 0, 0, 0, 0, 0, 0]
  set_cnt : Subsystem
  dout : Outport
  valid : Outport  Port=2
  wr_ack : Outport  Orientation=left  Port=3
  full : Outport  Port=4
  empty : Outport  Port=5
  wires:
  Delay1/1 -> valid/1
  Logical4/1 -> Delay1/1, rd_cnt/1
  re/1 -> Logical4/1
  Inverter1/1 -> Logical4/2
  Logical1/1 -> empty/1, Inverter1/1
  Dual Port RAM/2 -> dout/1
  Constant5/1 -> Dual Port RAM/6
  discard/1 -> set_cnt/2(undo)
  Logical3/1 -> set_cnt/3(en), Dual Port RAM/3, wr_ack/1
  we/1 -> Logical3/2
  Inverter2/1 -> Logical3/1, Logical1/2
  commit/1 -> set_cnt/1(set)
  rd_cnt/1 -> Slice/1, Slice1/1, Relational2/2
  set_cnt/1(set_cnt) -> Relational2/1
  set_cnt/2(cnt) -> Slice3/1, Slice2/1
  Slice/1 -> Dual Port RAM/4, Relational1/2
  din/1 -> Dual Port RAM/5, Dual Port RAM/2
  Slice2/1 -> Dual Port RAM/1, Relational1/1
  Slice3/1 -> Logical5/1
  Slice1/1 -> Logical5/2
  Relational1/1 -> Logical6/2
  Logical5/1 -> Logical6/1
  Logical6/1 -> full/1, Inverter2/1
  Relational2/1 -> Logical1/1

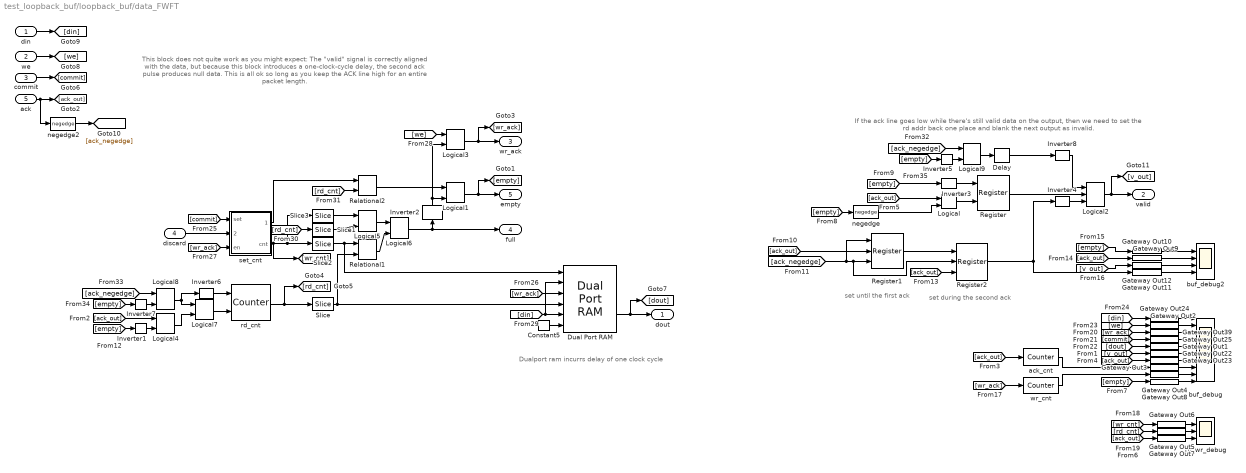
== system test_loopback_buf/loopback_buf/data_FWFT ==
  note: This block does not quite work as you might expect:
      | The "valid" signal is correctly aligned with the data,
      | but because this block introduces a one-clock-cycle delay,
      | the second ack pulse produces null data.
      |
      | This is all ok so long as you keep the ACK line high for an entire packet length.
  note: set until the first ack
  note: set during the second ack
  note: If the ack line goes low while there's still valid data on the output,
      | then we need to set the rd addr back one place and blank the next
      | output as invalid.
  note: Dualport ram incurrs delay
      | of one clock cycle
  din : Inport  Port=1  LatchInput=off
  we : Inport  Port=2  LatchInput=off
  commit : Inport  Port=3  LatchInput=off
  discard : Inport  Port=4  LatchInput=off
  ack : Inport  Port=5  LatchInput=off
  Constant5 : xbsIndex_r3/Constant  const=0  equ=P=C  arith_type=Boolean  n_bits=1  bin_pt=0  opselect=C  inp2=PCIN>>17  opr=+  inp1=P  carry=CIN  iostate=0  explicit_period=on  period=1  dbl_ovrd=off
  Delay : xbsIndex_r3/Delay  latency=1  reg_retiming=off  explicit_period=off  period=1  en=off  accept_only_valid=off  init_zero=on  dbl_ovrd=off  show_param=off
      settings: xl_area=[0, 0, 0, 0, 0, 0, 0]
  Dual Port RAM : xbsIndex_r3/Dual Port RAM  depth=2^depth_bits  initVector=0  write_mode_A=Read Before Write  write_mode_B=Read Before Write  latency=1  mem_collision=off  init_zero=on  explicit_period=off  period=1  dbl_ovrd=off  rst_a=off  init_a=0  rst_b=off  init_b=0  show_param=off  distributed_mem=off  use_rpm=off  gen_core=off
      settings: xl_area=[0, 0, 0, 0, 0, 0, 0]
  Gateway Out{1..12,22..25,39} (17 alike) : xbsIndex_r3/Gateway Out  output_type=Double  nbits=8  bin_pt=6  arith_type=Boolean  quantization=Truncate  overflow=Wrap  hdl_port=on  timing_constraint=None  locs_specified=off  LOCs={}  needs_fixed_name=off  show_param=off
      settings: xl_area=[0, 0, 0, 0, 0, 0, 0]
  Inverter{1,3..8} (7 alike) : xbsIndex_r3/Inverter  latency=0  explicit_period=off  period=1  en=off  dbl_ovrd=off  show_param=off
      settings: xl_area=[0, 0, 0, 0, 0, 0, 0]
  Inverter2 : xbsIndex_r3/Inverter  Orientation=up  latency=0  explicit_period=off  period=1  en=off  dbl_ovrd=off  show_param=off
      settings: xl_area=[0, 0, 0, 0, 0, 0, 0]
  Logical : xbsIndex_r3/Logical  logical_function=OR  inputs=2  precision=Full  arith_type=Unsigned  n_bits=8  bin_pt=2  align_bp=on  latency=0  explicit_period=off  period=1  en=off  dbl_ovrd=off  show_param=off
      settings: xl_area=[0, 0, 0, 0, 0, 0, 0]
  Logical1 : xbsIndex_r3/Logical  logical_function=AND  inputs=2  precision=Full  arith_type=Unsigned  n_bits=8  bin_pt=2  align_bp=on  latency=0  explicit_period=on  period=1  en=off  dbl_ovrd=off  show_param=off
      settings: xl_area=[0, 0, 0, 0, 0, 0, 0]
  Logical2 : xbsIndex_r3/Logical  logical_function=AND  inputs=3  precision=Full  arith_type=Unsigned  n_bits=8  bin_pt=2  align_bp=on  latency=0  explicit_period=on  period=1  en=off  dbl_ovrd=off  show_param=off
      settings: xl_area=[0, 0, 0, 0, 0, 0, 0]
  Logical{3..4,6,8..9} (5 alike) : xbsIndex_r3/Logical  logical_function=AND  inputs=2  precision=Full  arith_type=Unsigned  n_bits=8  bin_pt=2  align_bp=on  latency=0  explicit_period=off  period=1  en=off  dbl_ovrd=off  show_param=off
      settings: xl_area=[0, 0, 0, 0, 0, 0, 0]
  Logical5 : xbsIndex_r3/Logical  logical_function=XOR  inputs=2  precision=Full  arith_type=Unsigned  n_bits=8  bin_pt=2  align_bp=on  latency=0  explicit_period=off  period=1  en=off  dbl_ovrd=off  show_param=off
      settings: xl_area=[0, 0, 0, 0, 0, 0, 0]
  Logical7 : xbsIndex_r3/Logical  logical_function=OR  inputs=2  precision=Full  arith_type=Unsigned  n_bits=8  bin_pt=2  align_bp=on  latency=0  explicit_period=off  period=1  en=off  dbl_ovrd=off  show_param=off
      settings: xl_area=[0, 0, 0, 0, 0, 0, 0]
  Register : xbsIndex_r3/Register  init=0  reg_only_valid=off  explicit_period=on  period=1  rst=off  en=on  out_en=off  dbl_ovrd=off  show_param=off
      settings: xl_area=[0, 0, 0, 0, 0, 0, 0]
  Register1 : xbsIndex_r3/Register  init=0  reg_only_valid=off  explicit_period=on  period=1  rst=on  en=on  out_en=off  dbl_ovrd=off  show_param=off
      settings: xl_area=[0, 0, 0, 0, 0, 0, 0]
  Register2 : xbsIndex_r3/Register  init=0  reg_only_valid=off  explicit_period=on  period=1  rst=on  en=on  out_en=off  dbl_ovrd=off  show_param=off
      settings: xl_area=[0, 0, 0, 0, 0, 0, 0]
  Relational1 : xbsIndex_r3/Relational  mode=a=b  latency=0  explicit_period=on  period=1  en=off  dbl_ovrd=off  show_param=off
      settings: xl_area=[0, 0, 0, 0, 0, 0, 0]
  Relational2 : xbsIndex_r3/Relational  mode=a=b  latency=0  explicit_period=on  period=1  en=off  dbl_ovrd=off  show_param=off
      settings: xl_area=[0, 0, 0, 0, 0, 0, 0]
  Slice : xbsIndex_r3/Slice  mode=Two Bit Locations  nbits=1  bit1=-1  base1=MSB of Input  bit0=0  base0=LSB of Input  boolean_output=off  explicit_period=off  period=1  dbl_ovrd=off
  Slice1 : xbsIndex_r3/Slice  mode=Upper Bit Location + Width  nbits=1  bit1=0  base1=MSB of Input  bit0=0  base0=LSB of Input  boolean_output=on  explicit_period=off  period=1  dbl_ovrd=off
  Slice2 : xbsIndex_r3/Slice  mode=Two Bit Locations  nbits=1  bit1=-1  base1=MSB of Input  bit0=0  base0=LSB of Input  boolean_output=off  explicit_period=off  period=1  dbl_ovrd=off
  Slice3 : xbsIndex_r3/Slice  mode=Upper Bit Location + Width  nbits=1  bit1=0  base1=MSB of Input  bit0=0  base0=LSB of Input  boolean_output=on  explicit_period=off  period=1  dbl_ovrd=off
  ack_cnt : xbsIndex_r3/Counter  cnt_type=Free Running  n_bits=depth_bits + 1  bin_pt=0  arith_type=Unsigned  start_count=0  cnt_to=Inf  cnt_by_val=1  operation=Up  explicit_period=on  period=1  load_pin=off  rst=off  en=on  dbl_ovrd=off  show_param=off  use_rpm=on  gen_core=off
      settings: xl_area=[0, 0, 0, 0, 0, 0, 0]
  buf_debug : Scope  NumInputPorts=10
      settings: YMin=12000~0~9500~0~15500~-5~-5~-5~-5~-5  YMax=13300~1~10500~1~17250~5~5~5~5~5  SaveName=ScopeData13
  buf_debug2 : Scope  NumInputPorts=4
      settings: YMin=0~1~0~-1  YMax=1~1~1~1  SaveName=ScopeData15
  negedge : casper_library/Misc/negedge  Tag=Rising Edge Detector
  negedge2 : casper_library/Misc/negedge  Tag=Rising Edge Detector
  rd_cnt : xbsIndex_r3/Counter  cnt_type=Free Running  n_bits=depth_bits + 1  bin_pt=0  arith_type=Unsigned  start_count=0  cnt_to=Inf  cnt_by_val=1  operation=Up/Down  explicit_period=on  period=1  load_pin=off  rst=off  en=on  dbl_ovrd=off  show_param=off  use_rpm=on  gen_core=off
      settings: xl_area=[0, 0, 0, 0, 0, 0, 0]
  rd_wr_debug : Scope  NumInputPorts=3
      settings: YMin=12000~0~-5  YMax=13300~1~5  SaveName=ScopeData14
  set_cnt : Subsystem
  wr_cnt : xbsIndex_r3/Counter  cnt_type=Free Running  n_bits=depth_bits + 1  bin_pt=0  arith_type=Unsigned  start_count=0  cnt_to=Inf  cnt_by_val=1  operation=Up  explicit_period=on  period=1  load_pin=off  rst=off  en=on  dbl_ovrd=off  show_param=off  use_rpm=on  gen_core=off
      settings: xl_area=[0, 0, 0, 0, 0, 0, 0]
  dout : Outport
  valid : Outport  Port=2
  wr_ack : Outport  Port=3
  full : Outport  Port=4
  empty : Outport  Port=5
  wires:
  Relational2/1 -> Logical1/1
  Logical6/1 -> Inverter2/1, full/1
  Logical5/1 -> Logical6/1
  Relational1/1 -> Logical6/2
  Slice1/1 -> Logical5/2
  Slice3/1 -> Logical5/1
  Slice2/1 -> Relational1/1, Dual Port RAM/1
  Slice/1 -> Relational1/2, Dual Port RAM/4
  set_cnt/2(cnt) -> Slice3/1, Slice2/1, [wr_cnt]
  set_cnt/1(set_cnt) -> Relational2/1
  rd_cnt/1 -> [rd_cnt], Slice/1
  commit/1 -> [commit]
  Inverter2/1 -> Logical1/2, Logical3/2
  we/1 -> [we]
  discard/1 -> set_cnt/2(undo)
  Constant5/1 -> Dual Port RAM/6
  Dual Port RAM/2 -> dout/1, [dout]
  Logical1/1 -> [empty], empty/1
  Gateway Out24/1 -> buf_debug/1
  Gateway Out2/1 -> buf_debug/2
  Gateway Out39/1 -> buf_debug/3
  Gateway Out25/1 -> buf_debug/4
  Gateway Out1/1 -> buf_debug/5
  Gateway Out22/1 -> buf_debug/6
  Gateway Out23/1 -> buf_debug/7
  Gateway Out3/1 -> buf_debug/8
  Gateway Out4/1 -> buf_debug/9
  ack_cnt/1 -> Gateway Out3/1
  wr_cnt/1 -> Gateway Out4/1
  [empty] -> Inverter1/1
  [v_out] -> Gateway Out22/1
  ack/1 -> [ack_out], negedge2/1
  [ack_out] -> Logical4/1
  [ack_out] -> ack_cnt/1
  [ack_out] -> Gateway Out23/1
  Gateway Out6/1 -> rd_wr_debug/1
  Gateway Out5/1 -> rd_wr_debug/2
  Gateway Out7/1 -> rd_wr_debug/3
  [ack_out] -> Gateway Out7/1
  Gateway Out8/1 -> buf_debug/10
  [empty] -> Gateway Out8/1
  Inverter1/1 -> Logical4/2
  Logical2/1 -> valid/1, [v_out]
  [ack_negedge] -> Register1/1, Register1/3, Register2/2
  [ack_out] -> Register1/2
  Register1/1 -> Register2/1
  Gateway Out10/1 -> buf_debug2/1
  Gateway Out9/1 -> buf_debug2/2
  Gateway Out12/1 -> buf_debug2/3
  Gateway Out11/1 -> buf_debug2/4
  [ack_out] -> Gateway Out9/1
  [empty] -> Gateway Out10/1
  [v_out] -> Gateway Out12/1
  [ack_out] -> Register2/3
  [wr_ack] -> wr_cnt/1
  [wr_cnt] -> Gateway Out6/1
  [rd_cnt] -> Gateway Out5/1
  [wr_ack] -> Gateway Out39/1
  [commit] -> Gateway Out25/1
  [dout] -> Gateway Out1/1
  [we] -> Gateway Out2/1
  [din] -> Gateway Out24/1
  [commit] -> set_cnt/1(set)
  [wr_ack] -> Dual Port RAM/3
  [wr_ack] -> set_cnt/3(en)
  [we] -> Logical3/1
  Logical3/1 -> wr_ack/1, [wr_ack]
  [din] -> Dual Port RAM/2, Dual Port RAM/5
  din/1 -> [din]
  [rd_cnt] -> Slice1/1
  [rd_cnt] -> Relational2/2
  Register2/1 -> Gateway Out11/1, Inverter4/1
  negedge2/1 -> [ack_negedge]
  Inverter6/1 -> rd_cnt/1
  Logical7/1 -> rd_cnt/2
  Logical4/1 -> Logical7/2
  Logical8/1 -> Inverter6/1, Logical7/1
  [ack_negedge] -> Logical8/1
  [empty] -> Inverter7/1
  Inverter7/1 -> Logical8/2
  [ack_negedge] -> Logical9/1
  [empty] -> Inverter5/1
  Inverter5/1 -> Logical9/2
  Logical9/1 -> Delay/1
  Delay/1 -> Inverter8/1
  Inverter3/1 -> Register/1
  [empty] -> Inverter3/1
  Logical/1 -> Register/2
  [empty] -> negedge/1
  [ack_out] -> Logical/1
  negedge/1 -> Logical/2
  Inverter4/1 -> Logical2/3
  Inverter8/1 -> Logical2/1
  Register/1 -> Logical2/2
